simulink model "Rastrigin"  (R2019a)
settings: Solver=FixedStepAuto  StartTime=0.0  StopTime=size(InputValues_20200610T231852540,1) - 1  FixedStep=1  RelTol=1e-3
model workspace (MAT data in the model file):
  InputValues_20200610T231852540 = [0 0.0245361328125 0.049072265625 0.0736083984375 0.09814453125 0.122680664062 0.147216796875 0.171752929688 0.1962890625 0.220825195312 0.245361328125 0.269897460938 ... (257 elements, 257x1)]
libraries: simulink x1
settings Model: OrderedModelArguments=off  Creator=letras  LastModifiedBy=letras
settings DebuggingCC: IntegerOverflowMsg=none  ParameterOverflowMsg=none  ParameterPrecisionLossMsg=none  IntegerSaturationMsg=none

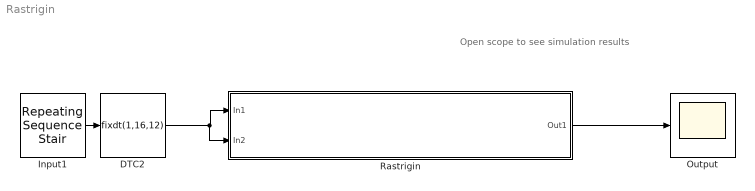
== system Rastrigin ==
  note: Open scope to see simulation results
  DTC2 : DataTypeConversion  OutDataTypeStr=fixdt(1,16,12)  RndMeth=Nearest
  Input1 : simulink/Sources/Repeating Sequence Stair  OutValues=[-5.12 -5 -4.5 -4.12 -3.12 -2.12 -1.12 0 1.12 2.12 3.12 4.12 5.12]  tsamp=-1  OutMin=[]  OutMax=[]  OutDataTypeStr=double  OutputDataTypeScalingMode=double  OutDataType=fixdt(0,8)  ConRadixGroup=Best Precision: Vector-wise  OutScaling=2^-12
  Output : Scope
  Rastrigin : Subsystem  Description=This block was created using function approximation.
  wires:
  Rastrigin/1(Out1) -> Output/1
  Input1/1 -> DTC2/1
  DTC2/1 -> Rastrigin/2(In2), Rastrigin/1(In1)

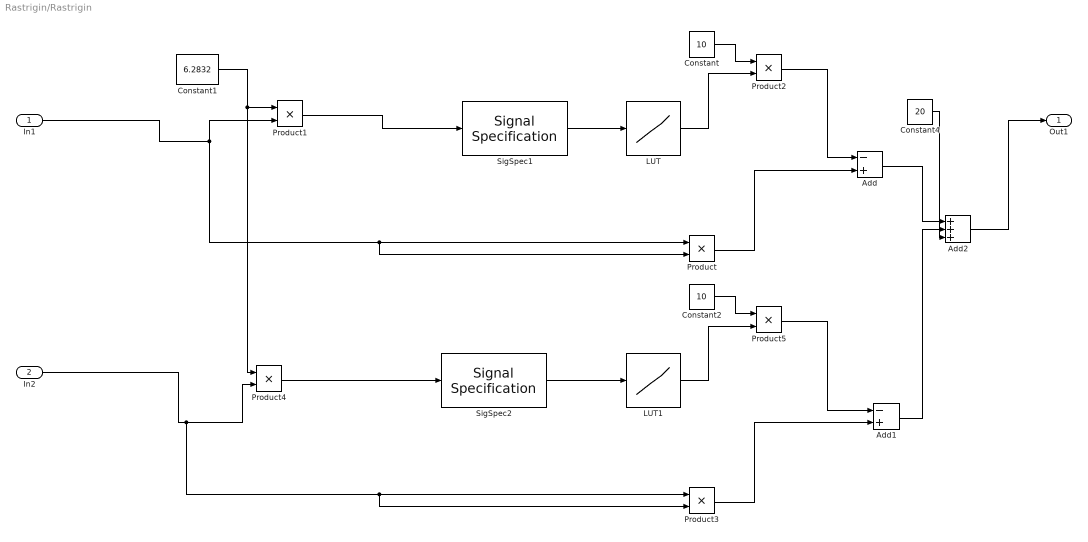
== system Rastrigin/Rastrigin ==
  In1 : Inport
  In2 : Inport  Port=2
  Add : Sum  Inputs=-+  OutDataTypeStr=fixdt(1,16,6)
  Add1 : Sum  Inputs=-+  OutDataTypeStr=fixdt(1,16,6)
  Add2 : Sum  Inputs=+++  OutDataTypeStr=fixdt(1,16,5)
  Constant : Constant  Value=10  OutDataTypeStr=fixdt(0,16,10)
  Constant1 : Constant  Value=6.2832  OutDataTypeStr=fixdt(0,16,12)
  Constant2 : Constant  Value=10  OutDataTypeStr=fixdt(0,16,10)
  Constant4 : Constant  Value=20  OutDataTypeStr=fixdt(0,16,5)
  LUT : Lookup_n-D  NumberOfTableDimensions=1  LookupTableObject=FunctionApproximation_LUTObject_20210714T214041645  BreakpointsSpecification=Even spacing  BreakpointsForDimension3=[5, 7]  BreakpointsForDimension1FirstPoint=-32.171875  BreakpointsForDimension1Spacing=1.00390625  BreakpointsForDimension1DataTypeStr=numerictype(1,16,9)  IndexSearchMethod=Evenly spaced points  Table=[0.72760009765625 0.96942138671875 0.31353759765625 -0.63262939453125 -0.9930419921875 -0.43389892578125 0.52703857421875 0.99993896484375 0.54693603515625 -0.41253662109375 -0.989990234375 -0.6507568359375 0.29107666015625 0.96337890625 0.74359130859375 -0.16473388671875 -0.9205322265625 -0.82391357421875 0.03558349609375 0.8621826171875 0.890380859375 0.0941162109375 -0.789306640625 -0.94183349609375 -0.2222900390625 0.703125 0.9774169921875 0.3466796875 -0.6051025390625 -0.99658203125 -0.4652099609375 0.49688720703125 0.9989013671875 0.575927734375 -0.38031005859375 -0.98443603515625 -0.67694091796875 0.25732421875 0.953369140625 0.7666015625 -0.1300048828125 -0.90625 -0.84332275390625 0.00054931640625 0.8438720703125 0.90582275390625 0.12896728515625 -0.76727294921875 -0.95306396484375 -0.25634765625 0.677734375 0.9842529296875 0.37933349609375 -0.5767822265625 -0.99884033203125 -0.4959716796875 0.46612548828125 0.99664306640625 0.604248046875 -0.34765625 -0.9776611328125 -0.702392578125 0.2232666015625 0.94219970703125 0.78863525390625]  TableDataTypeStr=numerictype(1,16,14)  ExtrapMethod=Clip  UseLastTableValue=on  InternalRulePriority=Speed  OutDataTypeStr=numerictype(1,16,14)  RndMeth=Simplest
  LUT1 : Lookup_n-D  NumberOfTableDimensions=1  LookupTableObject=FunctionApproximation_LUTObject_20210714T214041645  BreakpointsSpecification=Even spacing  BreakpointsForDimension3=[5, 7]  BreakpointsForDimension1FirstPoint=-32.171875  BreakpointsForDimension1Spacing=1.00390625  BreakpointsForDimension1DataTypeStr=numerictype(1,16,9)  IndexSearchMethod=Evenly spaced points  Table=[0.72760009765625 0.96942138671875 0.31353759765625 -0.63262939453125 -0.9930419921875 -0.43389892578125 0.52703857421875 0.99993896484375 0.54693603515625 -0.41253662109375 -0.989990234375 -0.6507568359375 0.29107666015625 0.96337890625 0.74359130859375 -0.16473388671875 -0.9205322265625 -0.82391357421875 0.03558349609375 0.8621826171875 0.890380859375 0.0941162109375 -0.789306640625 -0.94183349609375 -0.2222900390625 0.703125 0.9774169921875 0.3466796875 -0.6051025390625 -0.99658203125 -0.4652099609375 0.49688720703125 0.9989013671875 0.575927734375 -0.38031005859375 -0.98443603515625 -0.67694091796875 0.25732421875 0.953369140625 0.7666015625 -0.1300048828125 -0.90625 -0.84332275390625 0.00054931640625 0.8438720703125 0.90582275390625 0.12896728515625 -0.76727294921875 -0.95306396484375 -0.25634765625 0.677734375 0.9842529296875 0.37933349609375 -0.5767822265625 -0.99884033203125 -0.4959716796875 0.46612548828125 0.99664306640625 0.604248046875 -0.34765625 -0.9776611328125 -0.702392578125 0.2232666015625 0.94219970703125 0.78863525390625]  TableDataTypeStr=numerictype(1,16,14)  ExtrapMethod=Clip  UseLastTableValue=on  InternalRulePriority=Speed  OutDataTypeStr=numerictype(1,16,14)  RndMeth=Simplest
  Product : Product  OutDataTypeStr=fixdt(0,16,9)
  Product1 : Product  OutDataTypeStr=fixdt(1,16,9)
  Product2 : Product  OutDataTypeStr=fixdt(1,16,6)
  Product3 : Product  OutDataTypeStr=fixdt(0,16,9)
  Product4 : Product  OutDataTypeStr=fixdt(1,16,9)
  Product5 : Product  OutDataTypeStr=fixdt(1,16,6)
  SigSpec1 : SignalSpecification  OutMin=0  OutMax=1  OutDataTypeStr=numerictype(1,16,9)
  SigSpec2 : SignalSpecification  OutMin=0  OutMax=1  OutDataTypeStr=numerictype(1,16,9)
  Out1 : Outport
  wires:
  SigSpec1/1 -> LUT/1
  Constant1/1 -> Product4/1, Product1/1
  In1/1 -> Product1/2, Product/2, Product/1
  Constant/1 -> Product2/1
  LUT/1 -> Product2/2
  Product2/1 -> Add/1
  Constant2/1 -> Product5/1
  Product3/1 -> Add1/2
  LUT1/1 -> Product5/2
  SigSpec2/1 -> LUT1/1
  In2/1 -> Product4/2, Product3/2, Product3/1
  Product5/1 -> Add1/1
  Add2/1 -> Out1/1
  Add/1 -> Add2/1
  Add1/1 -> Add2/2
  Constant4/1 -> Add2/3
  Product/1 -> Add/2
  Product1/1 -> SigSpec1/1
  Product4/1 -> SigSpec2/1
